simulink model "FOC_IM_Reg_mech"  (R2018b)
settings: Solver=ode45  StartTime=0.0  StopTime=12  MaxStep=1e-6  RelTol=1e-6
values from neighbouring files (symbols this model uses):
  Af = 0.5    [Motor_parameters_project.m]
  Cd = 0.8    [Motor_parameters_project.m]
  density = 1.225    [Motor_parameters_project.m]
  fs = 10000    [Motor_parameters_project.m]
  g = 9.81    [Motor_parameters_project.m]
  Gr = 1.6666    [Motor_parameters_project.m]
  In = 189    [Motor_parameters_project.m]
  J = 0.0151    [Motor_parameters_project.m]
  Jw = 0.5*(Rw/Gr)^2*Mw    (= 0.0680679453267)    [Motor_parameters_project.m]
  Ki_d = 6.81    [Motor_parameters_project.m]
  Ki_q = 6.81    [Motor_parameters_project.m]
  Ki_speed = 0.35542    [Motor_parameters_project.m]
  Kp_d = 1.12    [Motor_parameters_project.m]
  Kp_q = 1.12    [Motor_parameters_project.m]
  Kp_speed = 3.5542    [Motor_parameters_project.m]
  landa_r = 0.0567    [Motor_parameters_project.m]
  Lm = 0.38e-3    (= 0.00038)    [Motor_parameters_project.m]
  Lr = Lm + Ldr    (= 0.00041116)    [Motor_parameters_project.m]
  Ls = Lm + Lds    (= 0.00041116)    [Motor_parameters_project.m]
  Mcar = 233    [Motor_parameters_project.m]
  p = 2.0    (= 2)    [Motor_parameters_project.m]
  Rr = 2.69e-3    (= 0.00269)    [Motor_parameters_project.m]
  Rs = 2.5e-3    (= 0.0025)    [Motor_parameters_project.m]
  Rw = 0.1375    [Motor_parameters_project.m]
  Ts = 1/fs    (= 0.0001)    [Motor_parameters_project.m]
  Udc = 36    [Motor_parameters_project.m]
  Un = 24/sqrt(3)    [Motor_parameters_project.m]
undefined symbols (not defined in the file or in its folder): DiscIntNeverNeededParam, magnitude, plecs, sigbuilder_block
libraries: dspsigops x1, powerlib x1
settings Model: Creator=estef  LastModifiedBy=faheem
settings DebuggingCC: MaxConsecutiveZCsMsg=warning

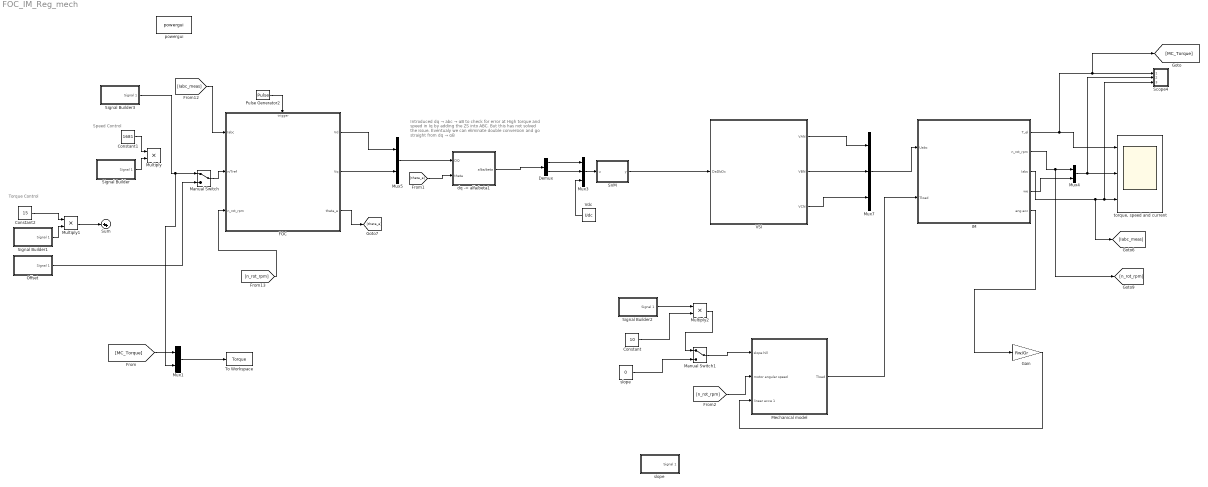
== system FOC_IM_Reg_mech ==
  note: Introduced dq → abc → αB to check for error at High
      | torque and speed in Iq by adding the ZS into ABC.
      | But this has not solved the issue. Eventualy we can
      | eliminate double conversion and go straight from dq → αB
  note: Speed Control
  note: Torque Control
  Constant : Constant  Value=10
  Constant1 : Constant  Value=1681
  Constant2 : Constant  Value=15
  Demux : Demux  Outputs=2
  "FOC " : Subsystem
  Gain : Gain  Gain=Rw/Gr
  "IM " : Subsystem
  Manual Switch : ManualSwitch
  Manual Switch1 : ManualSwitch
  "Mechanical model " : Subsystem
  Multiply : Product
  Multiply1 : Product
  Multiply2 : Product
  Mux1 : Mux  Inputs=2
  Mux3 : Mux  Inputs=3
  Mux4 : Mux  Inputs=2
  Mux5 : Mux  Inputs=2
  Mux7 : Mux  Inputs=3
  "Offset " : Subsystem  Tag=STV Subsys  LoadFcn=sigbuilder_block('load');  StartFcn=sigbuilder_block('start');  StopFcn=sigbuilder_block('stop');  ClipboardFcn=sigbuilder_block('clipboard');  mask(Sigbuilder block){tuvar=[0:10]}
      mask help: Simulink:masks:SigbuilderBlock_MD
      mask init:
      | if ~strcmp(get_param(bdroot(gcbh),'SimulationStatus'),'stopped') tuvar = sigbuilder_block('maskInit'); end
      settings: CopyFcn=sigbuilder_block('copy');  DeleteFcn=sigbuilder_block('delete');  ModelCloseFcn=sigbuilder_block('modelClose');  PreSaveFcn=sigbuilder_block('preSave');  PauseFcn=sigbuilder_block('pause');  ContinueFcn=sigbuilder_block('continue');  NameChangeFcn=sigbuilder_block('namechange');  OpenFcn=sigbuilder_block('open',[0 36 1280 617 ]);  CloseFcn=sigbuilder_block('close');
      mask Display: plot(0, 0, 100, 100,[2, 2, 32, 32, 2], [68, 8, 8, 68, 68],[32, 2], [38, 38], [32, 19, 2],[53, 60, 44], [32, 17, 17, 2],[16, 16, 31, 31]);txt = getActiveGroup(gcbh);text(2, 100, txt,'verticalAlignment', 'top');
  Pulse Generator2 : DiscretePulseGenerator  PulseType=Time based  Period=1/fs  PulseWidth=50
  SVM : MATLAB Function  TreatAsAtomicUnit=on
  Scope4 : Subsystem  LoadFcn=plecs('sl', 300);  InitFcn=plecs('sl', 314);  StartFcn=plecs('sl', 308);  StopFcn=plecs('sl', 309);  mask{Settings=}
      mask init:
      | plecs('sl', 315);
      settings: CopyFcn=plecs('sl', 303);  DeleteFcn=plecs('sl', 305);  UndoDeleteFcn=plecs('sl', 306);  PreSaveFcn=plecs('sl', 311);  NameChangeFcn=plecs('sl', 310);  DestroyFcn=plecs('sl', 307);  OpenFcn=plecs('sl', 302);  ErrorFcn=plerrorfcn
      mask Display: plot([0.1 0.9 0.9 0.1 0.1], [0.9 0.9 0.5 0.5 0.9])
  Signal Builder : Subsystem  Tag=STV Subsys  LoadFcn=sigbuilder_block('load');  StartFcn=sigbuilder_block('start');  StopFcn=sigbuilder_block('stop');  ClipboardFcn=sigbuilder_block('clipboard');  mask(Sigbuilder block){tuvar=[0:10]}
      mask help: Simulink:masks:SigbuilderBlock_MD
      mask init:
      | if ~strcmp(get_param(bdroot(gcbh),'SimulationStatus'),'stopped') tuvar = sigbuilder_block('maskInit'); end
      settings: CopyFcn=sigbuilder_block('copy');  DeleteFcn=sigbuilder_block('delete');  ModelCloseFcn=sigbuilder_block('modelClose');  PreSaveFcn=sigbuilder_block('preSave');  PauseFcn=sigbuilder_block('pause');  ContinueFcn=sigbuilder_block('continue');  NameChangeFcn=sigbuilder_block('namechange');  OpenFcn=sigbuilder_block('open',[534 149 550 400 ]);  CloseFcn=sigbuilder_block('close');
      mask Display: plot(0, 0, 100, 100,[2, 2, 32, 32, 2], [68, 8, 8, 68, 68],[32, 2], [38, 38], [32, 19, 2],[53, 60, 44], [32, 17, 17, 2],[16, 16, 31, 31]);txt = getActiveGroup(gcbh);text(2, 100, txt,'verticalAlignment', 'top');
  Signal Builder1 : Subsystem  Tag=STV Subsys  LoadFcn=sigbuilder_block('load');  StartFcn=sigbuilder_block('start');  StopFcn=sigbuilder_block('stop');  ClipboardFcn=sigbuilder_block('clipboard');  mask(Sigbuilder block){tuvar=[0:10]}
      mask help: Simulink:masks:SigbuilderBlock_MD
      mask init:
      | if ~strcmp(get_param(bdroot(gcbh),'SimulationStatus'),'stopped') tuvar = sigbuilder_block('maskInit'); end
      settings: CopyFcn=sigbuilder_block('copy');  DeleteFcn=sigbuilder_block('delete');  ModelCloseFcn=sigbuilder_block('modelClose');  PreSaveFcn=sigbuilder_block('preSave');  PauseFcn=sigbuilder_block('pause');  ContinueFcn=sigbuilder_block('continue');  NameChangeFcn=sigbuilder_block('namechange');  OpenFcn=sigbuilder_block('open',[19.8 157.8 550.2 400.2 ]);  CloseFcn=sigbuilder_block('close');
      mask Display: plot(0, 0, 100, 100,[2, 2, 32, 32, 2], [68, 8, 8, 68, 68],[32, 2], [38, 38], [32, 19, 2],[53, 60, 44], [32, 17, 17, 2],[16, 16, 31, 31]);txt = getActiveGroup(gcbh);text(2, 100, txt,'verticalAlignment', 'top');
  Signal Builder2 : Subsystem  Tag=STV Subsys  LoadFcn=sigbuilder_block('load');  StartFcn=sigbuilder_block('start');  StopFcn=sigbuilder_block('stop');  ClipboardFcn=sigbuilder_block('clipboard');  mask(Sigbuilder block){tuvar=[0:10]}
      mask help: Simulink:masks:SigbuilderBlock_MD
      mask init:
      | if ~strcmp(get_param(bdroot(gcbh),'SimulationStatus'),'stopped') tuvar = sigbuilder_block('maskInit'); end
      settings: CopyFcn=sigbuilder_block('copy');  DeleteFcn=sigbuilder_block('delete');  ModelCloseFcn=sigbuilder_block('modelClose');  PreSaveFcn=sigbuilder_block('preSave');  PauseFcn=sigbuilder_block('pause');  ContinueFcn=sigbuilder_block('continue');  NameChangeFcn=sigbuilder_block('namechange');  OpenFcn=sigbuilder_block('open',[334 138 550 400 ]);  CloseFcn=sigbuilder_block('close');
      mask Display: plot(0, 0, 100, 100,[2, 2, 32, 32, 2], [68, 8, 8, 68, 68],[32, 2], [38, 38], [32, 19, 2],[53, 60, 44], [32, 17, 17, 2],[16, 16, 31, 31]);txt = getActiveGroup(gcbh);text(2, 100, txt,'verticalAlignment', 'top');
  Signal Builder3 : Subsystem  Tag=STV Subsys  LoadFcn=sigbuilder_block('load');  StartFcn=sigbuilder_block('start');  StopFcn=sigbuilder_block('stop');  ClipboardFcn=sigbuilder_block('clipboard');  mask(Sigbuilder block){tuvar=[0:10]}
      mask help: Simulink:masks:SigbuilderBlock_MD
      mask init:
      | if ~strcmp(get_param(bdroot(gcbh),'SimulationStatus'),'stopped') tuvar = sigbuilder_block('maskInit'); end
      settings: CopyFcn=sigbuilder_block('copy');  DeleteFcn=sigbuilder_block('delete');  ModelCloseFcn=sigbuilder_block('modelClose');  PreSaveFcn=sigbuilder_block('preSave');  PauseFcn=sigbuilder_block('pause');  ContinueFcn=sigbuilder_block('continue');  NameChangeFcn=sigbuilder_block('namechange');  OpenFcn=sigbuilder_block('open',[437.6 199.2 550.4 400 ]);  CloseFcn=sigbuilder_block('close');
      mask Display: plot(0, 0, 100, 100,[2, 2, 32, 32, 2], [68, 8, 8, 68, 68],[32, 2], [38, 38], [32, 19, 2],[53, 60, 44], [32, 17, 17, 2],[16, 16, 31, 31]);txt = getActiveGroup(gcbh);text(2, 100, txt,'verticalAlignment', 'top');
  Sum : Sum  Inputs=|++
  To Workspace : ToWorkspace  VariableName=Torque  SaveFormat=Timeseries  SampleTime=-1
  VSI : Subsystem
  Vdc : Constant  Value=Udc
  "dq -> alfa/beta1" : Subsystem  mask(DQ -> ABC){}
      mask help: Implements DQ -> ABC transformation
      mask Display: disp(' ')
  powergui : powerlib/powergui  Priority=1  SimulationMode=Continuous  SampleTime=50e-6  frequency=60  Iterations=50  frequencyindice=60  Pbase=100e6  ErrMax=1e-4  UnitsV=kV  UnitsW=MW  buscounter=0  FunctionMessages=off  echomessages=off  EnableUseOfTLC=off  CurrentSourceSwitches=off  DisableSnubberDevices=off  DisableRonSwitches=off  DisableVfSwitches=off  DisplayEquations=off  SolverType=Tustin/Backward Euler (TBE)  Interpol=off  ExternalGateDelay=off  methode=off  Ts=100  x0status=blocks  SPID=on  SwTol=0  HookPort=off  RestoreLinks=warning  ResistiveCurrentMeasurement=off  Frange=[0:2:500]  Ylog=off  Xlog=on  ShowGrid=off  save=off  variable=ZData  structure=Sig1_Uabc_input  ZoomFFT=off  StartTime=0.3  cycles=10  DisplayStyle=1  fundamental=54  FreqAxis=off  MaxFrequency=1000  frequencyindicesteady=1  RmsSteady=1  display=off
  slope : Constant  Value=0
  "slope " : Subsystem  Tag=STV Subsys  LoadFcn=sigbuilder_block('load');  StartFcn=sigbuilder_block('start');  StopFcn=sigbuilder_block('stop');  ClipboardFcn=sigbuilder_block('clipboard');  mask(Sigbuilder block){tuvar=[0:10]}
      mask help: Simulink:masks:SigbuilderBlock_MD
      mask init:
      | if ~strcmp(get_param(bdroot(gcbh),'SimulationStatus'),'stopped') tuvar = sigbuilder_block('maskInit'); end
      settings: CopyFcn=sigbuilder_block('copy');  DeleteFcn=sigbuilder_block('delete');  ModelCloseFcn=sigbuilder_block('modelClose');  PreSaveFcn=sigbuilder_block('preSave');  PauseFcn=sigbuilder_block('pause');  ContinueFcn=sigbuilder_block('continue');  NameChangeFcn=sigbuilder_block('namechange');  OpenFcn=sigbuilder_block('open',[730 198 550 298 ]);  CloseFcn=sigbuilder_block('close');
      mask Display: plot(0, 0, 100, 100,[2, 2, 32, 32, 2], [68, 8, 8, 68, 68],[32, 2], [38, 38], [32, 19, 2],[53, 60, 44], [32, 17, 17, 2],[16, 16, 31, 31]);txt = getActiveGroup(gcbh);text(2, 100, txt,'verticalAlignment', 'top');
  "torque, speed and current " : Scope  NumInputPorts=3
  wires:
  Mux7/1 -> "IM "/1("Uabc ")
  VSI/3(VCN) -> Mux7/3
  "IM "/1(T_el) -> Scope4/1(1), [MC_Torque], "torque, speed and current "/1
  VSI/1("VAN ") -> Mux7/1
  VSI/2("VBN ") -> Mux7/2
  "IM "/3(Iabc) -> [Iabc_meas], Scope4/3(3), "torque, speed and current "/3
  "FOC "/1(Vd) -> Mux5/1
  [Iabc_meas] -> "FOC "/1("Iabc ")
  "FOC "/2("Vq ") -> Mux5/2
  [n_rot_rpm] -> "FOC "/3("n_rot_rpm ")
  Manual Switch/1 -> "FOC "/2(n/Tref)
  "FOC "/3("theta_e ") -> [theta_e]
  Mux4/1 -> Scope4/2(2), "torque, speed and current "/2
  "IM "/2("n_rot_rpm ") -> [n_rot_rpm], Mux4/1
  Demux/2 -> Mux3/2
  Mux3/1 -> SVM/1(u)
  Demux/1 -> Mux3/1
  SVM/1(y) -> VSI/1(DaDbDc)
  Vdc/1 -> Mux3/3
  Mux5/1 -> "dq -> alfa/beta1"/1(DQ)
  "dq -> alfa/beta1"/1(alba/beta) -> Demux/1
  [theta_e] -> "dq -> alfa/beta1"/2(theta)
  Multiply1/1 -> Sum/1
  Constant2/1 -> Multiply1/1
  Signal Builder/1(Signal 1) -> Multiply/2
  Constant1/1 -> Multiply/1
  Signal Builder1/1(Signal 1) -> Multiply1/2
  "IM "/4("we ") -> Mux4/2
  Pulse Generator2/1 -> "FOC "/Trigger
  Constant/1 -> Multiply2/2
  "Mechanical model "/1(Tload) -> "IM "/2("Tload ")
  Manual Switch1/1 -> "Mechanical model "/1("slope hill ")
  [n_rot_rpm] -> "Mechanical model "/2("motor angular speed ")
  "Offset "/1(Signal 1) -> Manual Switch/2
  Multiply2/1 -> Manual Switch1/1
  "IM "/5("ang acc ") -> Gain/1
  Gain/1 -> "Mechanical model "/3(linear acce 1)
  slope/1 -> Manual Switch1/2
  Signal Builder3/1(Signal 1) -> Mux1/2, Manual Switch/1
  Signal Builder2/1(Signal 1) -> Multiply2/1
  [MC_Torque] -> Mux1/1
  Mux1/1 -> To Workspace/1

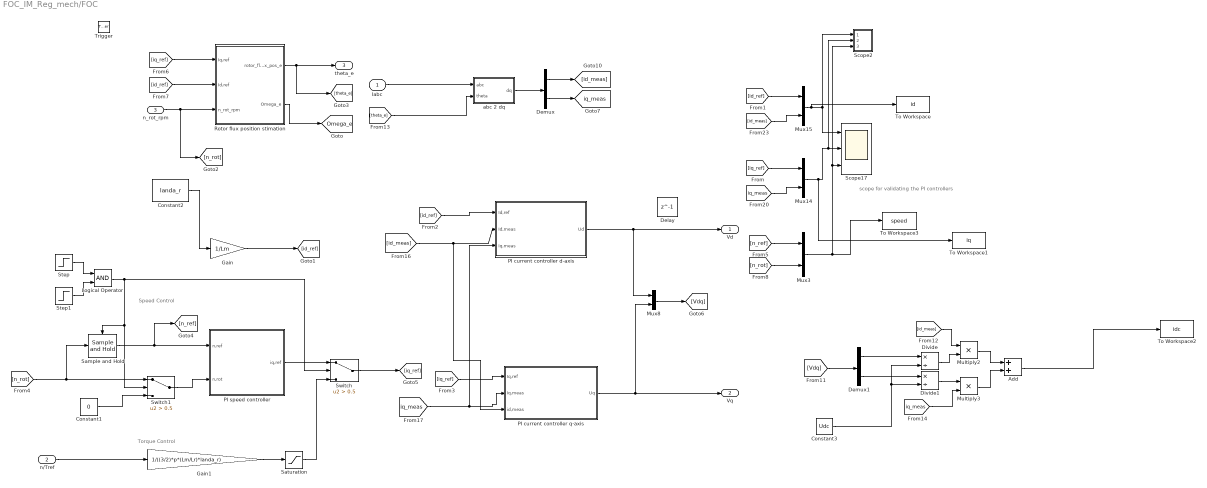
== system FOC_IM_Reg_mech/FOC  ==
  note: Speed Control
  note: scope for validating the PI controllers
  note: Torque Control
  "Iabc " : Inport
  n/Tref : Inport  Port=2
  "n_rot_rpm " : Inport  Port=3
  Trigger : TriggerPort  VariantControl=Variant  PortDimensions=1
  Add : Sum
  Constant1 : Constant  Value=0
  Constant2 : Constant  Value=landa_r
  Constant3 : Constant  Value=Udc
  Delay : Delay  DelayLength=1
  Demux : Demux  Outputs=2
  Demux1 : Demux  Outputs=2
  Divide : Product  Inputs=*/
  Divide1 : Product  Inputs=*/
  Gain : Gain  Gain=1/Lm
  Gain1 : Gain  Gain=1/((3/2)*p*(Lm/Lr)*landa_r)
  Logical Operator : Logic  AllPortsSameDT=off  OutDataTypeStr=boolean
  Multiply2 : Product
  Multiply3 : Product
  Mux{3,8,14..15} (4 alike) : Mux  Inputs=2
  PI current controller d-axis : Subsystem
  PI current controller q-axis : Subsystem
  PI speed controller : Subsystem
  Rotor flux position stimation : Subsystem
  Sample and Hold : dspsigops/Sample and Hold  trig=Rising edge  initCond=0  latchinput=off
  Saturation : Saturate  UpperLimit=In*sqrt(2)  LowerLimit=-In*sqrt(2)
  Scope17 : Scope  NumInputPorts=3
  Scope2 : Subsystem  LoadFcn=plecs('sl', 300);  InitFcn=plecs('sl', 314);  StartFcn=plecs('sl', 308);  StopFcn=plecs('sl', 309);  mask{Settings=}
      mask init:
      | plecs('sl', 315);
      settings: CopyFcn=plecs('sl', 303);  DeleteFcn=plecs('sl', 305);  UndoDeleteFcn=plecs('sl', 306);  PreSaveFcn=plecs('sl', 311);  NameChangeFcn=plecs('sl', 310);  DestroyFcn=plecs('sl', 307);  OpenFcn=plecs('sl', 302);  ErrorFcn=plerrorfcn
      mask Display: plot([0.1 0.9 0.9 0.1 0.1], [0.9 0.9 0.5 0.5 0.9])
  Step : Step  Time=7.5
  Step1 : Step  Time=11  Before=1  After=0
  Switch : Switch  Criteria=u2 > Threshold  Threshold=0.5
  Switch1 : Switch  Criteria=u2 > Threshold  Threshold=0.5
  To Workspace : ToWorkspace  VariableName=id  SaveFormat=Timeseries  SampleTime=-1
  To Workspace1 : ToWorkspace  VariableName=iq  SaveFormat=Timeseries  SampleTime=-1
  To Workspace2 : ToWorkspace  VariableName=idc  SaveFormat=Timeseries  SampleTime=-1
  To Workspace3 : ToWorkspace  VariableName=speed  SaveFormat=Timeseries  SampleTime=-1
  abc 2 dq : Subsystem
  Vd : Outport
  "Vq " : Outport  Port=2
  "theta_e " : Outport  Port=3
  tag scope: Omega_e=global, iq_meas=global
  wires:
  Mux15/1 -> To Workspace/1, Scope2/1(1), Scope17/1
  [id_meas] -> Mux15/2
  [iq_meas] -> Mux14/2
  Demux/2 -> [iq_meas]
  [theta_e] -> abc 2 dq/2(theta)
  abc 2 dq/1(dq) -> Demux/1
  Demux/1 -> [id_meas]
  [iq_ref] -> Mux14/1
  [id_ref] -> Mux15/1
  Mux14/1 -> To Workspace1/1, Scope2/2(2), Scope17/2
  [id_meas] -> PI current controller q-axis/3("id,meas "), PI current controller d-axis/2(Id,meas)
  [iq_meas] -> PI current controller d-axis/3("Iq,meas "), PI current controller q-axis/2(Iq,meas)
  Rotor flux position stimation/1(rotor_flux_pos_e) -> [theta_e], "theta_e "/1
  [iq_ref] -> Rotor flux position stimation/1(Iq,ref)
  [id_ref] -> Rotor flux position stimation/2(Id,ref)
  "n_rot_rpm "/1 -> [n_rot], Rotor flux position stimation/3(n_rot_rpm)
  Gain/1 -> [id_ref]
  [n_ref] -> Mux3/1
  [n_rot] -> Mux3/2
  Mux3/1 -> To Workspace3/1, Scope2/3(3), Scope17/3
  [id_ref] -> PI current controller d-axis/1(Id,ref)
  [iq_ref] -> PI current controller q-axis/1("Iq,ref ")
  "Iabc "/1 -> abc 2 dq/1(abc)
  Step/1 -> Logical Operator/1
  Step1/1 -> Logical Operator/2
  Logical Operator/1 -> Switch/2, Switch1/2, Sample and Hold/Trigger
  Gain1/1 -> Saturation/1
  Rotor flux position stimation/2(Omega_e) -> [Omega_e]
  [Vdq] -> Demux1/1
  Demux1/1 -> Divide/1
  Constant3/1 -> Divide1/2, Divide/2
  Demux1/2 -> Divide1/1
  [id_meas] -> Multiply2/1
  Divide/1 -> Multiply2/2
  Divide1/1 -> Multiply3/1
  [iq_meas] -> Multiply3/2
  Multiply2/1 -> Add/1
  Multiply3/1 -> Add/2
  Add/1 -> To Workspace2/1
  PI current controller q-axis/1("Uq ") -> "Vq "/1, Mux8/2
  PI current controller d-axis/1(Ud) -> Vd/1, Mux8/1
  Constant2/1 -> Gain/1
  Saturation/1 -> Switch/3
  [n_rot] -> Switch1/1, Sample and Hold/1
  Mux8/1 -> [Vdq]
  n/Tref/1 -> Gain1/1
  Sample and Hold/1 -> [n_ref], PI speed controller/1(n,ref)
  PI speed controller/1("iq,ref ") -> Switch/1
  Switch/1 -> [iq_ref]
  Switch1/1 -> PI speed controller/2("n,rot ")
  Constant1/1 -> Switch1/3

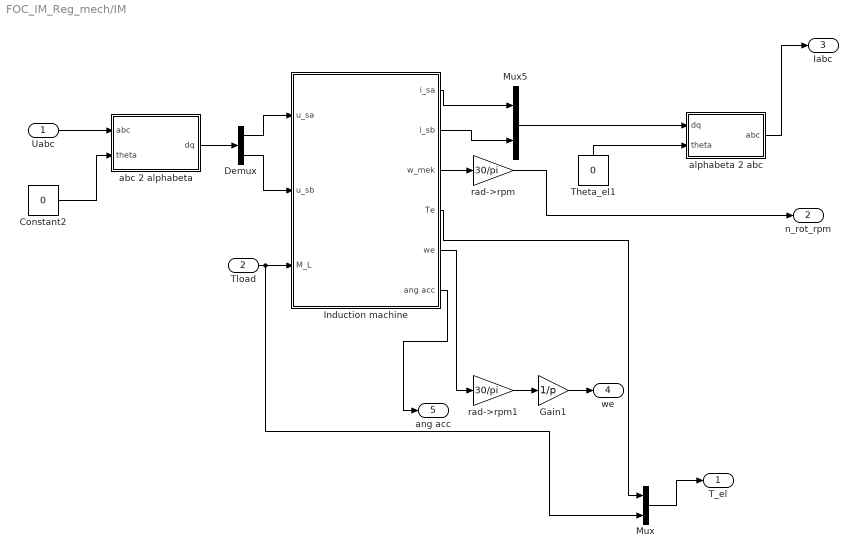
== system FOC_IM_Reg_mech/IM  ==
  "Uabc " : Inport
  "Tload " : Inport  Port=2
  Constant2 : Constant  Value=0
  Demux : Demux  Outputs=2
  Gain1 : Gain  Gain=1/p
  "Induction machine " : Subsystem
  Mux : Mux  Inputs=2
  Mux5 : Mux  Inputs=2
  Theta_el1 : Constant  Value=0
  abc 2 alphabeta : Subsystem
  alphabeta 2 abc : Subsystem
  rad->rpm : Gain  Gain=30/pi  SaturateOnIntegerOverflow=on  OutDataTypeStr=Inherit: Same as input  ParamDataTypeStr=Inherit: Same as input
  rad->rpm1 : Gain  Gain=30/pi  SaturateOnIntegerOverflow=on  OutDataTypeStr=Inherit: Same as input  ParamDataTypeStr=Inherit: Same as input
  T_el : Outport
  "n_rot_rpm " : Outport  Port=2
  Iabc : Outport  Port=3
  "we " : Outport  Port=4
  "ang acc " : Outport  Port=5
  wires:
  rad->rpm/1 -> "n_rot_rpm "/1
  "Induction machine "/4(Te) -> Mux/1
  Constant2/1 -> abc 2 alphabeta/2(theta)
  abc 2 alphabeta/1(dq) -> Demux/1
  Theta_el1/1 -> alphabeta 2 abc/2(theta)
  Mux5/1 -> alphabeta 2 abc/1(dq)
  "Induction machine "/1(i_sa) -> Mux5/1
  "Induction machine "/3(w_mek) -> rad->rpm/1
  "Induction machine "/2(i_sb) -> Mux5/2
  Demux/1 -> "Induction machine "/1(u_sa)
  Demux/2 -> "Induction machine "/2(u_sb)
  "Uabc "/1 -> abc 2 alphabeta/1(abc)
  alphabeta 2 abc/1(abc) -> Iabc/1
  "Induction machine "/5("we ") -> rad->rpm1/1
  rad->rpm1/1 -> Gain1/1
  Gain1/1 -> "we "/1
  "Tload "/1 -> Mux/2, "Induction machine "/3(M_L)
  Mux/1 -> T_el/1
  "Induction machine "/6("ang acc ") -> "ang acc "/1

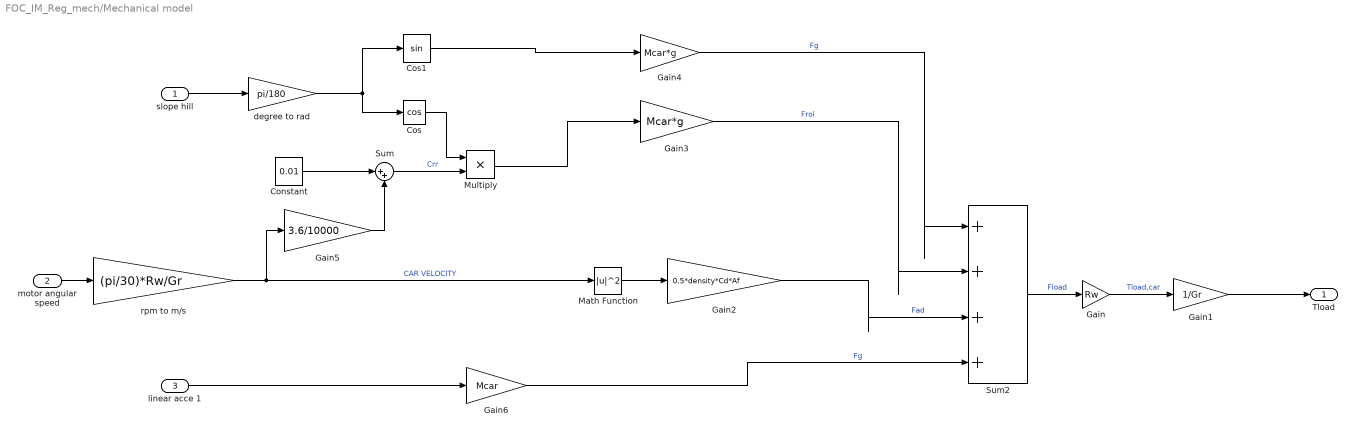
== system FOC_IM_Reg_mech/Mechanical model  ==
  "slope hill " : Inport
  "motor angular speed " : Inport  Port=2
  linear acce 1 : Inport  Port=3
  Constant : Constant  Value=0.01
  Cos : Trigonometry  Operator=cos
  Cos1 : Trigonometry
  Gain : Gain  Gain=Rw
  Gain1 : Gain  Gain=1/Gr
  Gain2 : Gain  Gain=0.5*density*Cd*Af
  Gain3 : Gain  Gain=Mcar*g
  Gain4 : Gain  Gain=Mcar*g
  Gain5 : Gain  Gain=3.6/10000
  Gain6 : Gain  Gain=Mcar
  Math Function : Math  Operator=magnitude^2  SaturateOnIntegerOverflow=on
  Multiply : Product
  Sum : Sum  Inputs=|++
  Sum2 : Sum  Inputs=|++++
  "degree to rad " : Gain  Gain=pi/180
  rpm to m/s : Gain  Gain=(pi/30)*Rw/Gr
  Tload : Outport
  wires:
  Cos1/1 -> Gain4/1
  Gain1/1 -> Tload/1
  Gain4/1 -> Sum2/1  "Fg"
  "degree to rad "/1 -> Cos/1, Cos1/1
  rpm to m/s/1 -> Math Function/1, Gain5/1  "CAR VELOCITY"
  Gain2/1 -> Sum2/3  "Fad"
  Math Function/1 -> Gain2/1
  "slope hill "/1 -> "degree to rad "/1
  Sum2/1 -> Gain/1  "Fload"
  Gain3/1 -> Sum2/2  "Frol"
  Gain/1 -> Gain1/1  "Tload,car"
  "motor angular speed "/1 -> rpm to m/s/1
  Constant/1 -> Sum/1
  Gain5/1 -> Sum/2
  Sum/1 -> Multiply/2  "Crr"
  Cos/1 -> Multiply/1
  Multiply/1 -> Gain3/1
  Gain6/1 -> Sum2/4  "Fg"
  linear acce 1/1 -> Gain6/1

== system FOC_IM_Reg_mech/Offset  ==
  Demux : Demux  Tag=STV Demux  Outputs=1
  FromWs : FromWorkspace  Tag=STV FromWs  VariableName=tuvar  SampleTime=0
      SigBuilderData=|
      | common.afterFinalStr = 'Extrapolate'
      | common.sampleTime = '0'
      | dataSet.timeRange = [0 2]
      | dataSet.name = 'Group 1'
      | sbobj.Groups.Name = 'Group 1'
      | sbobj.Groups.Signals.Name = 'Signal 1'
      | sbobj.Groups.Signals.XData = [0 0.2 0.405 0.6 0.66 0.8 0.92 1.2 1.57 1.624 2]
      | sbobj.Groups.Signals.YData = [0 20 30 28 -15.4 30 30 -30 -16.2 15 16.2]
      | sbobj.Groups.TimeRange = [0 2]
  Signal 1 : Outport  Tag=STV Outport
  wires:
  Demux/1 -> Signal 1/1
  FromWs/1 -> Demux/1

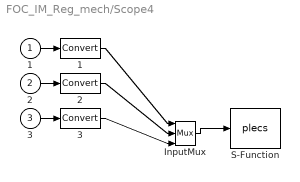
== system FOC_IM_Reg_mech/Scope4 ==
  1 : Inport
  2 : Inport  Port=2
  3 : Inport  Port=3
  " 1 " : DataTypeConversion  SaturateOnIntegerOverflow=on  RndMeth=Zero
  " 2 " : DataTypeConversion  SaturateOnIntegerOverflow=on  RndMeth=Zero
  " 3 " : DataTypeConversion  SaturateOnIntegerOverflow=on  RndMeth=Zero
  " InputMux " : Mux  Inputs=3
  " S-Function " : S-Function  FunctionName=plecs  SFunctionDeploymentMode=off  EnableBusSupport=off
  wires:
  " InputMux "/1 -> " S-Function "/1
  1/1 -> " 1 "/1
  " 1 "/1 -> " InputMux "/1
  2/1 -> " 2 "/1
  " 2 "/1 -> " InputMux "/2
  3/1 -> " 3 "/1
  " 3 "/1 -> " InputMux "/3

== system FOC_IM_Reg_mech/Signal Builder ==
  Demux : Demux  Tag=STV Demux  Outputs=1
  FromWs : FromWorkspace  Tag=STV FromWs  VariableName=tuvar  SampleTime=0
      SigBuilderData=|
      | common.afterFinalStr = 'Extrapolate'
      | common.sampleTime = '0'
      | dataSet.timeRange = [0 2]
      | dataSet.name = 'Group 1'
      | sbobj.Groups.Name = 'Group 1'
      | sbobj.Groups.Signals.Name = 'Signal 1'
      | sbobj.Groups.Signals.XData = [0 0.2 0.4 0.6 1.2 1.6 1.8 2]
      | sbobj.Groups.Signals.YData = [0 0.4 0.4 0.8 0.8 0.2 0.2 0]
      | sbobj.Groups.TimeRange = [0 2]
  Signal 1 : Outport  Tag=STV Outport
  wires:
  FromWs/1 -> Demux/1
  Demux/1 -> Signal 1/1

== system FOC_IM_Reg_mech/Signal Builder1 ==
  Demux : Demux  Tag=STV Demux  Outputs=1
  FromWs : FromWorkspace  Tag=STV FromWs  VariableName=tuvar  SampleTime=0
      SigBuilderData=|
      | common.afterFinalStr = 'Extrapolate'
      | common.sampleTime = '0'
      | dataSet.timeRange = [0 2]
      | dataSet.name = 'Group 1'
      | sbobj.Groups.Name = 'Group 1'
      | sbobj.Groups.Signals.Name = 'Signal 1'
      | sbobj.Groups.Signals.XData = [0 0.15 0.2 0.25 0.4 0.6 1 1.3 1.5 2]
      | sbobj.Groups.Signals.YData = [0.4 0.52 0.58 0.995 0.995 0.9 0.995 0.81 0.64 0.3]
      | sbobj.Groups.TimeRange = [0 2]
  Signal 1 : Outport  Tag=STV Outport
  wires:
  FromWs/1 -> Demux/1
  Demux/1 -> Signal 1/1

== system FOC_IM_Reg_mech/Signal Builder2 ==
  Demux : Demux  Tag=STV Demux  Outputs=1
  FromWs : FromWorkspace  Tag=STV FromWs  VariableName=tuvar  SampleTime=0
      SigBuilderData=|
      | common.afterFinalStr = 'Extrapolate'
      | common.sampleTime = 0
      | dataSet.timeRange = [0 12]
      | dataSet.name = 'Group 1'
      | sbobj.Groups.Name = 'Group 1'
      | sbobj.Groups.Signals.Name = 'Signal 1'
      | sbobj.Groups.Signals.XData = [0 2 8.5 9.5 10.5 12]
      | sbobj.Groups.Signals.YData = [0 -0.005 0 -1 0 0]
      | sbobj.Groups.TimeRange = [0 12]
  Signal 1 : Outport  Tag=STV Outport
  wires:
  Demux/1 -> Signal 1/1
  FromWs/1 -> Demux/1

== system FOC_IM_Reg_mech/Signal Builder3 ==
  Demux : Demux  Tag=STV Demux  Outputs=1
  FromWs : FromWorkspace  Tag=STV FromWs  VariableName=tuvar  SampleTime=0
      SigBuilderData=|
      | common.afterFinalStr = 'Extrapolate'
      | common.sampleTime = 0
      | dataSet.timeRange = [0 12]
      | dataSet.name = 'Group 1'
      | sbobj.Groups.Name = 'Group 1'
      | sbobj.Groups.Signals.Name = 'Signal 1'
      | sbobj.Groups.Signals.XData = [0 0.2 0.5 6 6.3 7 7.2 8.2 12]
      | sbobj.Groups.Signals.YData = [2 5 30.04 30 -30.04 -30.04 30.04 30.0316666667 30]
      | sbobj.Groups.TimeRange = [0 12]
  Signal 1 : Outport  Tag=STV Outport
  wires:
  Demux/1 -> Signal 1/1
  FromWs/1 -> Demux/1

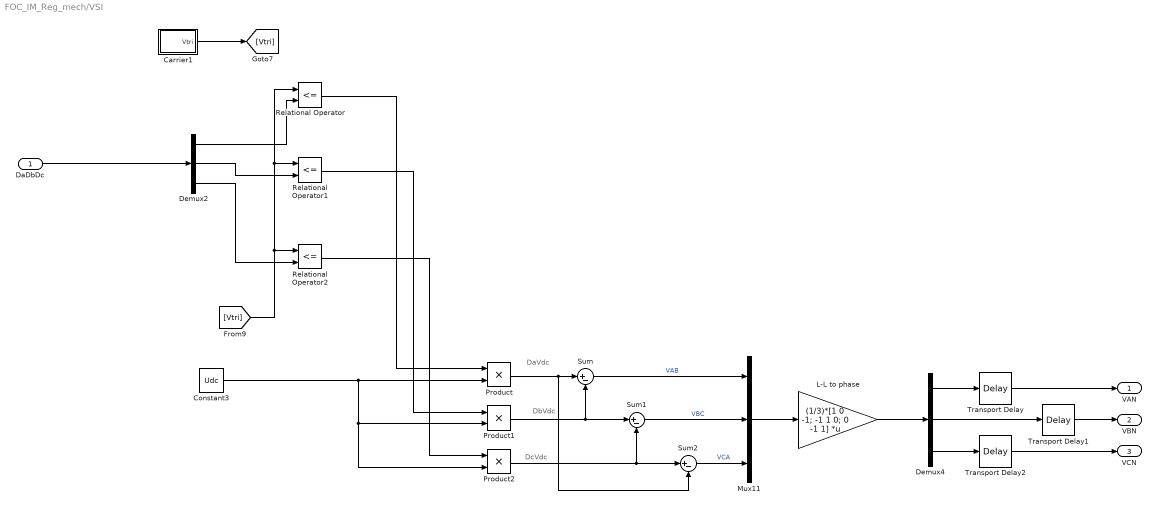
== system FOC_IM_Reg_mech/VSI ==
  note: DcVdc
  note: DaVdc
  note: DbVdc
  DaDbDc : Inport
  Carrier1 : Subsystem  mask{fsw=fs}
      mask prompts: fsw "switching frequency"
      mask init:
      | fsw2=fsw*2;
      | x=[0 1/4 3/4 1];
      | y=[0 -1     1    0];
      mask Display: plot([x  x+1 ],[y y])
  Constant3 : Constant  Value=Udc
  Demux2 : Demux  Outputs=3
  Demux4 : Demux  Outputs=3
  "L-L to phase " : Gain  Gain=(1/3)*[1 0 -1; -1 1 0; 0 -1 1]  Multiplication=Matrix(K*u)
  Mux11 : Mux  Inputs=3
  Product : Product
  Product1 : Product
  Product2 : Product
  Relational Operator : RelationalOperator  Operator=<=  OutDataTypeStr=boolean  ZeroCross=off  RndMeth=Simplest
  Relational Operator1 : RelationalOperator  Operator=<=  OutDataTypeStr=boolean  ZeroCross=off  RndMeth=Simplest
  Relational Operator2 : RelationalOperator  Operator=<=  OutDataTypeStr=boolean  ZeroCross=off  RndMeth=Simplest
  Sum : Sum  Inputs=|+-
  Sum1 : Sum  Inputs=|+-
  Sum2 : Sum  Inputs=|+-
  Transport Delay : TransportDelay  DelayTime=Ts/2
  Transport Delay1 : TransportDelay  DelayTime=Ts/2
  Transport Delay2 : TransportDelay  DelayTime=Ts/2
  "VAN " : Outport
  "VBN " : Outport  Port=2
  VCN : Outport  Port=3
  wires:
  Sum1/1 -> Mux11/2  "VBC"
  Carrier1/1(Vtri) -> [Vtri]
  Constant3/1 -> Product2/2, Product1/2, Product/2
  Demux2/2 -> Relational Operator1/2
  Product/1 -> Sum/1, Sum2/2
  [Vtri] -> Relational Operator1/1, Relational Operator/1, Relational Operator2/1
  Demux2/1 -> Relational Operator/2
  Relational Operator/1 -> Product/1
  Mux11/1 -> "L-L to phase "/1
  Product1/1 -> Sum1/1, Sum/2
  Product2/1 -> Sum2/1, Sum1/2
  Demux2/3 -> Relational Operator2/2
  Relational Operator2/1 -> Product2/1
  Sum/1 -> Mux11/1  "VAB"
  Sum2/1 -> Mux11/3  "VCA"
  Relational Operator1/1 -> Product1/1
  DaDbDc/1 -> Demux2/1
  "L-L to phase "/1 -> Demux4/1
  Demux4/2 -> Transport Delay1/1
  Demux4/3 -> Transport Delay2/1
  Demux4/1 -> Transport Delay/1
  Transport Delay/1 -> "VAN "/1
  Transport Delay1/1 -> "VBN "/1
  Transport Delay2/1 -> VCN/1

== system FOC_IM_Reg_mech/dq -> alfa//beta1 ==
  DQ : Inport
  theta : Inport  Port=2
  Mux : Mux  Inputs=[2 1]
  Mux1 : Mux  Inputs=2
  alfa-axis : Fcn  Expr=u[1]*cos(u[3])-u[2]*sin(u[3])
  beta-axis : Fcn  Expr=u[1]*sin(u[3])+u[2]*cos(u[3])
  alba/beta : Outport  InitialOutput=0
  wires:
  theta/1 -> Mux/2
  Mux1/1 -> alba/beta/1
  beta-axis/1 -> Mux1/2
  alfa-axis/1 -> Mux1/1
  DQ/1 -> Mux/1
  Mux/1 -> alfa-axis/1, beta-axis/1

== system FOC_IM_Reg_mech/slope  ==
  Demux : Demux  Tag=STV Demux  Outputs=1
  FromWs : FromWorkspace  Tag=STV FromWs  VariableName=tuvar  SampleTime=0
      SigBuilderData=|
      | common.afterFinalStr = 'Extrapolate'
      | common.sampleTime = '0'
      | dataSet.timeRange = [0 2]
      | dataSet.name = 'Group 1'
      | sbobj.Groups.Name = 'Group 1'
      | sbobj.Groups.Signals.Name = 'Signal 1'
      | sbobj.Groups.Signals.XData = [0 0.19 0.41 0.62 1 1.2 1.25 2]
      | sbobj.Groups.Signals.YData = [0 0 0 0 0 -1 0 0]
      | sbobj.Groups.TimeRange = [0 2]
  Signal 1 : Outport  Tag=STV Outport
  wires:
  FromWs/1 -> Demux/1
  Demux/1 -> Signal 1/1

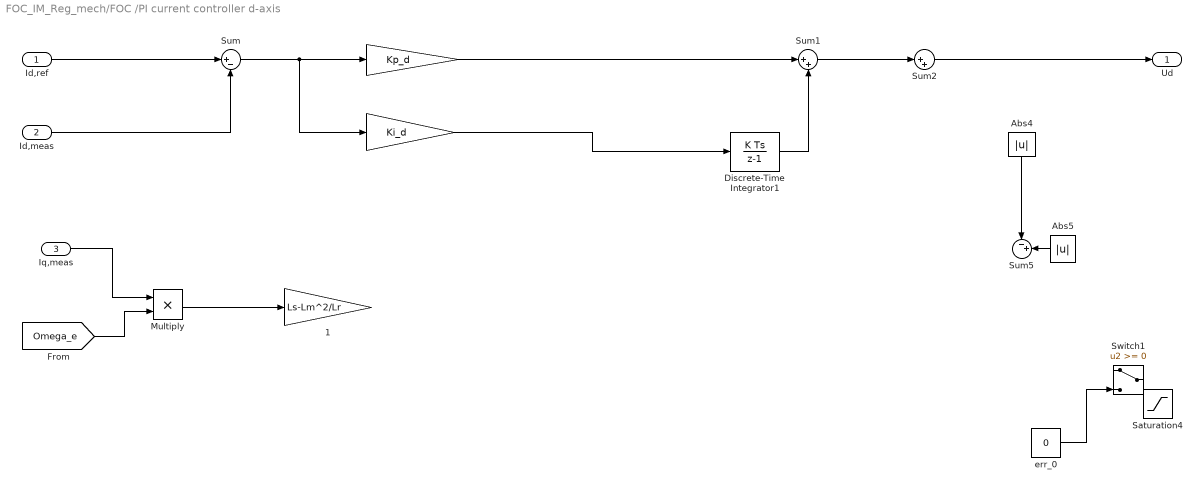
== system FOC_IM_Reg_mech/FOC /PI current controller d-axis ==
  Id,ref : Inport
  Id,meas : Inport  Port=2
  "Iq,meas " : Inport  Port=3
  "  " : Gain  Gain=Ki_d
  "   " : Gain  Gain=Kp_d
  "  1" : Gain  Gain=Ls-Lm^2/Lr
  Abs4 : Abs
  Abs5 : Abs
  Discrete-Time Integrator1 : DiscreteIntegrator  gainval=1  SampleTime=-1  UpperSaturationLimit=100  LowerSaturationLimit=-100  ICPrevOutput=DiscIntNeverNeededParam  ICPrevScaledInput=DiscIntNeverNeededParam
  Multiply : Product
  Saturation4 : Saturate  UpperLimit=Un*sqrt(2)  LowerLimit=-Un*sqrt(2)
  Sum : Sum  Inputs=|+-
  Sum1 : Sum  Inputs=|++
  Sum2 : Sum  Inputs=|++
  Sum5 : Sum  Inputs=-+|
  Switch1 : Switch
  err_0 : Constant  Value=0
  Ud : Outport
  wires:
  Id,ref/1 -> Sum/1
  Sum/1 -> "  "/1, "   "/1
  Id,meas/1 -> Sum/2
  err_0/1 -> Switch1/3
  Abs4/1 -> Sum5/1
  Abs5/1 -> Sum5/2
  Discrete-Time Integrator1/1 -> Sum1/2
  "   "/1 -> Sum1/1
  "  "/1 -> Discrete-Time Integrator1/1
  Sum1/1 -> Sum2/1
  "Iq,meas "/1 -> Multiply/1
  [Omega_e] -> Multiply/2
  Multiply/1 -> "  1"/1
  Sum2/1 -> Ud/1

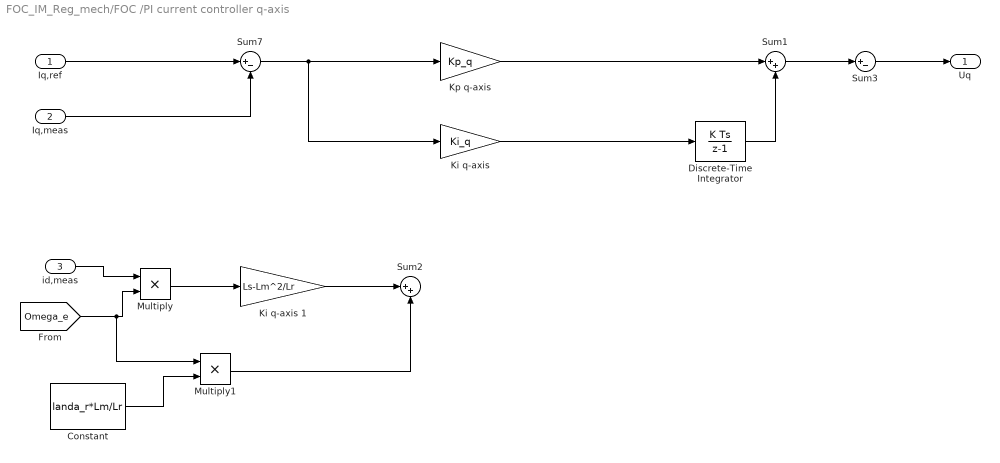
== system FOC_IM_Reg_mech/FOC /PI current controller q-axis ==
  "Iq,ref " : Inport
  Iq,meas : Inport  Port=2
  "id,meas " : Inport  Port=3
  Constant : Constant  Value=landa_r*Lm/Lr
  Discrete-Time Integrator : DiscreteIntegrator  gainval=1  SampleTime=-1  UpperSaturationLimit=100  LowerSaturationLimit=-100  ICPrevOutput=DiscIntNeverNeededParam  ICPrevScaledInput=DiscIntNeverNeededParam
  "Ki q-axis " : Gain  Gain=Ki_q
  Ki q-axis 1 : Gain  Gain=Ls-Lm^2/Lr
  Kp q-axis : Gain  Gain=Kp_q
  Multiply : Product
  Multiply1 : Product
  Sum1 : Sum  Inputs=|++
  Sum2 : Sum  Inputs=|++
  Sum3 : Sum  Inputs=|+-  SaturateOnIntegerOverflow=on  InputSameDT=on  OutDataTypeStr=Inherit: Same as first input
  Sum7 : Sum  Inputs=|+-  SaturateOnIntegerOverflow=on  InputSameDT=on  OutDataTypeStr=Inherit: Same as first input
  "Uq " : Outport
  wires:
  Sum7/1 -> "Ki q-axis "/1, Kp q-axis/1
  "Iq,ref "/1 -> Sum7/1
  Iq,meas/1 -> Sum7/2
  Kp q-axis/1 -> Sum1/1
  Discrete-Time Integrator/1 -> Sum1/2
  "Ki q-axis "/1 -> Discrete-Time Integrator/1
  "id,meas "/1 -> Multiply/1
  [Omega_e] -> Multiply1/1, Multiply/2
  Multiply/1 -> Ki q-axis 1/1
  Constant/1 -> Multiply1/2
  Ki q-axis 1/1 -> Sum2/1
  Multiply1/1 -> Sum2/2
  Sum1/1 -> Sum3/1
  Sum3/1 -> "Uq "/1

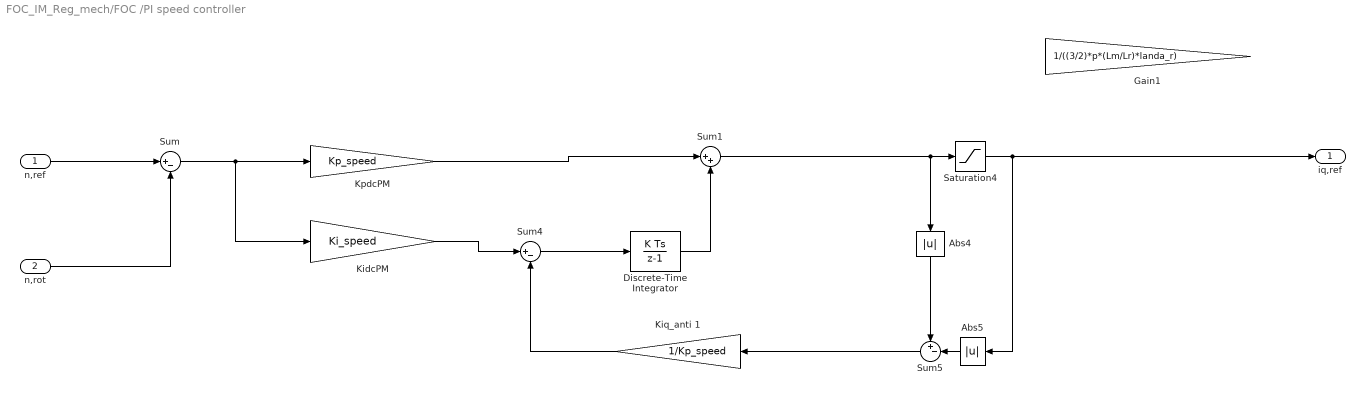
== system FOC_IM_Reg_mech/FOC /PI speed controller ==
  n,ref : Inport
  "n,rot " : Inport  Port=2
  Abs4 : Abs
  Abs5 : Abs
  Discrete-Time Integrator : DiscreteIntegrator  gainval=1  SampleTime=-1  UpperSaturationLimit=100  LowerSaturationLimit=-100  ICPrevOutput=DiscIntNeverNeededParam  ICPrevScaledInput=DiscIntNeverNeededParam
  Gain1 : Gain  Gain=1/((3/2)*p*(Lm/Lr)*landa_r)
  KidcPM : Gain  Gain=Ki_speed
  Kiq_anti 1 : Gain  Gain=1/Kp_speed
  KpdcPM : Gain  Gain=Kp_speed
  Saturation4 : Saturate  UpperLimit=In*sqrt(2)  LowerLimit=-In*sqrt(2)
  Sum : Sum  Inputs=|+-
  Sum1 : Sum  Inputs=|++
  Sum4 : Sum  Inputs=|+-
  Sum5 : Sum  Inputs=+-|
  "iq,ref " : Outport
  wires:
  Saturation4/1 -> "iq,ref "/1, Abs5/1
  Sum1/1 -> Abs4/1, Saturation4/1
  Abs5/1 -> Sum5/2
  KpdcPM/1 -> Sum1/1
  Abs4/1 -> Sum5/1
  KidcPM/1 -> Sum4/1
  n,ref/1 -> Sum/1
  "n,rot "/1 -> Sum/2
  Sum/1 -> KidcPM/1, KpdcPM/1
  Discrete-Time Integrator/1 -> Sum1/2
  Sum4/1 -> Discrete-Time Integrator/1
  Sum5/1 -> Kiq_anti 1/1
  Kiq_anti 1/1 -> Sum4/2

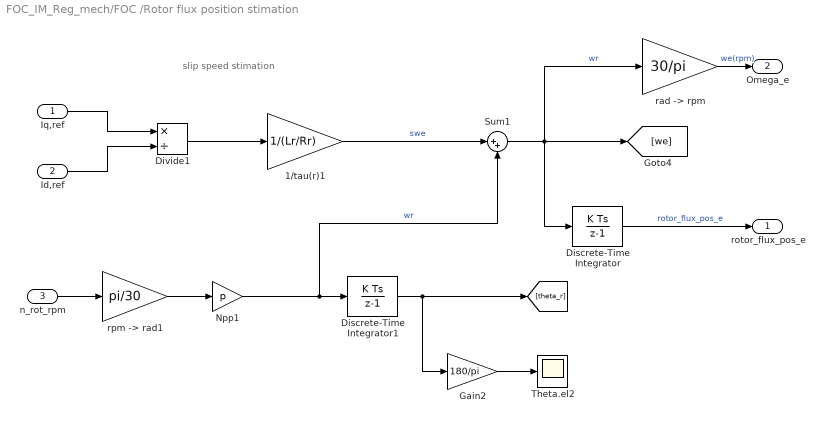
== system FOC_IM_Reg_mech/FOC /Rotor flux position stimation ==
  note: slip speed stimation
  Iq,ref : Inport
  Id,ref : Inport  Port=2
  n_rot_rpm : Inport  Port=3
  1/tau(r)1 : Gain  Gain=1/(Lr/Rr)
  Discrete-Time Integrator : DiscreteIntegrator  gainval=1  SampleTime=-1  UpperSaturationLimit=100  LowerSaturationLimit=-100  ICPrevOutput=DiscIntNeverNeededParam  ICPrevScaledInput=DiscIntNeverNeededParam
  Discrete-Time Integrator1 : DiscreteIntegrator  gainval=1  SampleTime=-1  UpperSaturationLimit=100  LowerSaturationLimit=-100  ICPrevOutput=DiscIntNeverNeededParam  ICPrevScaledInput=DiscIntNeverNeededParam
  Divide1 : Product  Inputs=*/
  Gain2 : Gain  Gain=180/pi
  Npp1 : Gain  Gain=p  SaturateOnIntegerOverflow=on  OutDataTypeStr=Inherit: Same as input  ParamDataTypeStr=Inherit: Same as input
  Sum1 : Sum  Inputs=|++
  Theta.el2 : Scope
  "rad -> rpm " : Gain  Gain=30/pi
  "rpm -> rad1" : Gain  Gain=pi/30  SaturateOnIntegerOverflow=on  OutDataTypeStr=Inherit: Same as input  ParamDataTypeStr=Inherit: Same as input
  rotor_flux_pos_e : Outport
  Omega_e : Outport  Port=2
  wires:
  Discrete-Time Integrator/1 -> rotor_flux_pos_e/1  "rotor_flux_pos_e"
  1/tau(r)1/1 -> Sum1/1  "swe"
  Npp1/1 -> Discrete-Time Integrator1/1, Sum1/2  "wr"
  "rpm -> rad1"/1 -> Npp1/1
  Iq,ref/1 -> Divide1/1
  Discrete-Time Integrator1/1 -> [theta_r], Gain2/1
  Divide1/1 -> 1/tau(r)1/1
  Gain2/1 -> Theta.el2/1
  n_rot_rpm/1 -> "rpm -> rad1"/1
  Id,ref/1 -> Divide1/2
  Sum1/1 -> "rad -> rpm "/1, Discrete-Time Integrator/1, [we]  "wr"
  "rad -> rpm "/1 -> Omega_e/1  "we(rpm)"

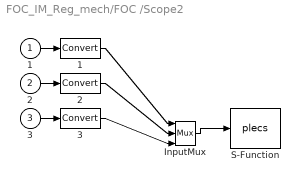
== system FOC_IM_Reg_mech/FOC /Scope2 ==
  1 : Inport
  2 : Inport  Port=2
  3 : Inport  Port=3
  " 1 " : DataTypeConversion  SaturateOnIntegerOverflow=on  RndMeth=Zero
  " 2 " : DataTypeConversion  SaturateOnIntegerOverflow=on  RndMeth=Zero
  " 3 " : DataTypeConversion  SaturateOnIntegerOverflow=on  RndMeth=Zero
  " InputMux " : Mux  Inputs=3
  " S-Function " : S-Function  FunctionName=plecs  SFunctionDeploymentMode=off  EnableBusSupport=off
  wires:
  " InputMux "/1 -> " S-Function "/1
  1/1 -> " 1 "/1
  " 1 "/1 -> " InputMux "/1
  2/1 -> " 2 "/1
  " 2 "/1 -> " InputMux "/2
  3/1 -> " 3 "/1
  " 3 "/1 -> " InputMux "/3

== system FOC_IM_Reg_mech/FOC /abc 2 dq ==
  abc : Inport
  theta : Inport  Port=2
  Mux1 : Mux  Inputs=2
  Mux2 : Mux  Inputs=2
  abc2d : Fcn  Expr=2/3*(u(1)*cos(u(4))+u(2)*cos(u(4)-2*pi/3)+u(3)*cos(u(4)-4*pi/3))
  abc2q : Fcn  Expr=-2/3*(u(1)*sin(u(4))+u(2)*sin(u(4)-2*pi/3)+u(3)*sin(u(4)-4*pi/3))
  dq : Outport
  wires:
  abc/1 -> Mux1/1
  theta/1 -> Mux1/2
  Mux1/1 -> abc2d/1, abc2q/1
  abc2d/1 -> Mux2/1
  abc2q/1 -> Mux2/2
  Mux2/1 -> dq/1

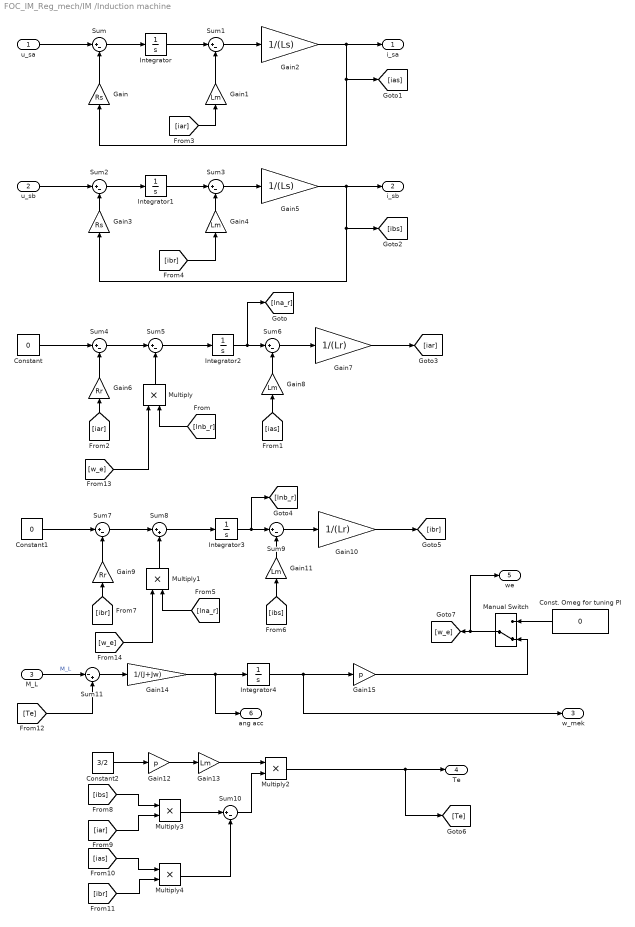
== system FOC_IM_Reg_mech/IM /Induction machine  ==
  u_sa : Inport
  u_sb : Inport  Port=2
  M_L : Inport  Port=3
  "Const. Omeg for tuning PI " : Constant  Value=0
  Constant : Constant  Value=0
  Constant1 : Constant  Value=0
  Constant2 : Constant  Value=3/2
  Gain : Gain  Gain=Rs
  Gain{1,4,8,11,13} (5 alike) : Gain  Gain=Lm
  Gain10 : Gain  Gain=1/(Lr)
  Gain12 : Gain  Gain=p
  Gain14 : Gain  Gain=1/(J+Jw)
  Gain15 : Gain  Gain=p
  Gain2 : Gain  Gain=1/(Ls)
  Gain3 : Gain  Gain=Rs
  Gain5 : Gain  Gain=1/(Ls)
  Gain6 : Gain  Gain=Rr
  Gain7 : Gain  Gain=1/(Lr)
  Gain9 : Gain  Gain=Rr
  Integrator{,1..4} (5 alike) : Integrator
  Manual Switch : ManualSwitch  CurrentSetting=0
  Multiply{,1..4} (5 alike) : Product
  Sum{,1..7,9..10} (10 alike) : Sum  Inputs=|+-
  Sum11 : Sum  Inputs=|-+
  Sum8 : Sum  Inputs=|++
  i_sa : Outport
  i_sb : Outport  Port=2
  w_mek : Outport  Port=3
  Te : Outport  Port=4
  "we " : Outport  Port=5
  "ang acc " : Outport  Port=6
  wires:
  u_sa/1 -> Sum/1
  Gain/1 -> Sum/2
  Sum/1 -> Integrator/1
  Integrator/1 -> Sum1/1
  Gain1/1 -> Sum1/2
  Sum1/1 -> Gain2/1
  Gain2/1 -> [ias], Gain/1, i_sa/1
  Gain3/1 -> Sum2/2
  u_sb/1 -> Sum2/1
  Sum3/1 -> Gain5/1
  Gain4/1 -> Sum3/2
  Gain5/1 -> i_sb/1, [ibs], Gain3/1
  Sum2/1 -> Integrator1/1
  Integrator1/1 -> Sum3/1
  Constant/1 -> Sum4/1
  Gain6/1 -> Sum4/2
  Sum4/1 -> Sum5/1
  [lnb_r] -> Multiply/2
  Sum5/1 -> Integrator2/1
  Gain8/1 -> Sum6/2
  [ias] -> Gain8/1
  Integrator2/1 -> [lna_r], Sum6/1
  Sum6/1 -> Gain7/1
  Multiply/1 -> Sum5/2
  Gain7/1 -> [iar]
  [iar] -> Gain6/1
  [ibr] -> Gain4/1
  [iar] -> Gain1/1
  Gain11/1 -> Sum9/2
  Gain10/1 -> [ibr]
  [ibr] -> Gain9/1
  [ibs] -> Gain11/1
  Multiply1/1 -> Sum8/2
  Integrator3/1 -> [lnb_r], Sum9/1
  Sum7/1 -> Sum8/1
  [lna_r] -> Multiply1/2
  Gain9/1 -> Sum7/2
  Sum9/1 -> Gain10/1
  Sum8/1 -> Integrator3/1
  Constant1/1 -> Sum7/1
  Gain13/1 -> Multiply2/1
  Sum10/1 -> Multiply2/2
  [ibs] -> Multiply3/1
  [iar] -> Multiply3/2
  Multiply3/1 -> Sum10/1
  [ias] -> Multiply4/1
  [ibr] -> Multiply4/2
  Multiply4/1 -> Sum10/2
  Constant2/1 -> Gain12/1
  Gain12/1 -> Gain13/1
  Multiply2/1 -> [Te], Te/1
  [Te] -> Sum11/2
  M_L/1 -> Sum11/1  "M_L"
  Sum11/1 -> Gain14/1
  Gain14/1 -> "ang acc "/1, Integrator4/1
  [w_e] -> Multiply/1
  [w_e] -> Multiply1/1
  "Const. Omeg for tuning PI "/1 -> Manual Switch/1
  Gain15/1 -> Manual Switch/2
  Manual Switch/1 -> "we "/1, [w_e]
  Integrator4/1 -> w_mek/1, Gain15/1

== system FOC_IM_Reg_mech/IM /abc 2 alphabeta ==
  abc : Inport
  theta : Inport  Port=2
  Mux1 : Mux  Inputs=2
  Mux2 : Mux  Inputs=2
  abc2d : Fcn  Expr=2/3*(u(1)*cos(u(4))+u(2)*cos(u(4)-2*pi/3)+u(3)*cos(u(4)-4*pi/3))
  abc2q : Fcn  Expr=-2/3*(u(1)*sin(u(4))+u(2)*sin(u(4)-2*pi/3)+u(3)*sin(u(4)-4*pi/3))
  dq : Outport
  wires:
  abc/1 -> Mux1/1
  theta/1 -> Mux1/2
  Mux1/1 -> abc2d/1, abc2q/1
  abc2d/1 -> Mux2/1
  abc2q/1 -> Mux2/2
  Mux2/1 -> dq/1

== system FOC_IM_Reg_mech/IM /alphabeta 2 abc ==
  dq : Inport
  theta : Inport  Port=2
  Mux1 : Mux  Inputs=2
  Mux2 : Mux  Inputs=3
  dq2a : Fcn  Expr=(cos(u(3))*u(1)-sin(u(3))*u(2))
  dq2b : Fcn  Expr=(cos(u(3)-2*pi/3)*u(1)-sin(u(3)-2*pi/3)*u(2))
  dq2c : Fcn  Expr=(cos(u(3)+2*pi/3)*u(1)-sin(u(3)+2*pi/3)*u(2))
  abc : Outport
  wires:
  Mux2/1 -> abc/1
  dq2b/1 -> Mux2/2
  dq2a/1 -> Mux2/1
  Mux1/1 -> dq2a/1, dq2c/1, dq2b/1
  theta/1 -> Mux1/2
  dq/1 -> Mux1/1
  dq2c/1 -> Mux2/3

== system FOC_IM_Reg_mech/VSI/Carrier1 ==
  note: set istart time 1/fsw/4
      | set initial IC 0.5
      | to have another waveform
      |  as shown on the block
  Constant : Constant
  Constant1 : Constant  Value=2*fs
  Integrator1 : Integrator
  Product : Product  SaturateOnIntegerOverflow=on  OutDataTypeStr=Inherit: Same as first input
  Pulse Generator : DiscretePulseGenerator  PulseType=Time based  Amplitude=2  Period=1/fsw  PulseWidth=50
  Sum : Sum  Inputs=|+-  SaturateOnIntegerOverflow=on
  Vtri : Outport  InitialOutput=0
  wires:
  Pulse Generator/1 -> Sum/1
  Constant/1 -> Sum/2
  Sum/1 -> Product/1
  Constant1/1 -> Product/2
  Product/1 -> Integrator1/1
  Integrator1/1 -> Vtri/1

== matlab function FOC_IM_Reg_mech/SVM ==
  data: u input; y output
function y = fcn(u)
% Space Vector Modulation

y                = zeros(3,1);

vsd              = u(1);  % V_alfa
vsq              = u(2);  % V_beta
Vdc              = u(3);  % DC link voltage 

% =========================================================================
% Set the voltage limits

weight           = Vdc/(sqrt(3)*sqrt(vsd*vsd+vsq*vsq));
dlimit           = abs(vsd*weight);
qlimit           = abs(vsq*weight);
if (abs(vsd)>dlimit)
    vsd          = (3*sign(vsd)*dlimit)/(2*Vdc);
else
    vsd          = (3*vsd)/(2*Vdc);
end

if(abs(vsq)>qlimit)
    vsq          = (3*sign(vsq)*qlimit)/(2*Vdc);
else
    vsq          = (3*vsq)/(2*Vdc);
end

duty_a           = 0;
duty_b           = 0;
duty_c           = 0;

% =========================================================================

if ((vsd>=0) && (vsq>=0)) 	
     if (vsq < sqrt(3)*vsd)
         % sector 0
         t1      = 0.5*(vsd-(vsq/sqrt(3)));
         t2      = vsq/sqrt(3);
         temp    = 0.5-t1-t2;
         duty_a  = 1-temp; 
         duty_b  = 1-(temp+2*t1);
         duty_c  = temp;
     else
         % sector 1
         t1      = 0.5*((vsq/sqrt(3))-vsd);
         t2      = 0.5*((vsq/sqrt(3))+vsd);
         temp    = 0.5-t1-t2;
         duty_b  = 1-temp; 
         duty_a  = 1-(temp+2*t1);
         duty_c  = temp;
     end
end

if ((vsd<0) && (vsq>0))
    if (vsq < (sqrt(3)*abs(vsd))) 
        % sector 2
        t1       = (vsq/sqrt(3));
        t2       = 0.5*(abs(vsd)-(vsq/sqrt(3)));
        temp     = 0.5-t1-t2;
        duty_b   = 1-temp; 		
        duty_c   = 1-(temp+2*t1);
        duty_a   = temp;
    else
        % sector 1
        t1       = 0.5*((vsq/sqrt(3))-vsd);
        t2       = 0.5*((vsq/sqrt(3))+vsd);
        temp     = 0.5-t1-t2;
        duty_b   = 1-temp; 	
        duty_a   = 1-(temp+2*t1);
        duty_c   = temp;
    end
end
       
if ((vsd<0) && (vsq<=0)) 	
    if (abs(vsq) <= sqrt(3)*abs(vsd)) 
        % Sector 3
        t1       = (abs(vsq)/sqrt(3));
        t2       = 0.5*(abs(vsd)-(abs(vsq)/sqrt(3)));
        temp     = 0.5-t1-t2;
        duty_c   = 1-temp; 			
        duty_b   = 1-(temp+2*t1);
        duty_a   = temp;
    else
        % Sector 4
        t1       = 0.5*((abs(vsq)/sqrt(3))-vsd);
        t2       = 0.5*((abs(vsq)/sqrt(3))+vsd);
        temp     = 0.5-t1-t2;
        duty_c   = 1-temp; 
        duty_a   = 1-(temp+2*t1);
        duty_b   = temp;
    end
end
   

if ((vsd>=0) && (vsq<0))	
    if(abs(vsq)<=vsd*sqrt(3))
        % Sector 5
        t1       = 0.5*(vsd-(abs(vsq)/sqrt(3)));
        t2       = (abs(vsq)/sqrt(3));
        temp     = 0.5-t1-t2;
        duty_a   = 1-temp; 				
        duty_c   = 1-(temp+2*t1);
        duty_b   = temp;
    else
        % Sector 4
        t1       = 0.5*((abs(vsq)/sqrt(3))-vsd);
        t2       = 0.5*((abs(vsq)/sqrt(3))+vsd);
        temp     = 0.5-t1-t2;
        duty_c   = 1-temp; 
        duty_a   = 1-(temp+2*t1);
        duty_b   = temp;
    end
end

% =========================================================================

y(1) = duty_a;
y(2) = duty_b;
y(3) = duty_c;

% =========================================================================
